simulink model "rtwdemo_capi"  (Simulink 7.6)
settings: Solver=FixedStepDiscrete  StartTime=0.0  StopTime=10.0  RelTol=1e-3  SampleTimeConstraint=STIndependent
PostLoadFcn:
  | rtwdemo_capi_data
values from neighbouring files (symbols this model uses):
  Kp = Simulink.Parameter    [rtwdemo_capi_data.m]
  p1 = Simulink.Parameter    [rtwdemo_capi_data.m]
  p2 = Simulink.Parameter    [rtwdemo_capi_data.m]
  p3 = Simulink.Parameter    [rtwdemo_capi_data.m]
libraries: rtwdemowidgets x2
Description:
  | Target-Based Data Interface: C-API Data Definition File
settings Model: Creator=The MathWorks Inc.  ExtModeTrigMode=oneshot  ExtModeArmWhenConnect=off  ExtModeAutoUpdateStatusClock=off
settings DataIOCC: LimitDataPoints=off  SaveFormat=Structure  SaveOutput=off  SaveTime=off  SignalLoggingName=sigsOut
settings OptimizationCC: InlineParams=on  InlineInvariantSignals=on  StateBitsets=on  DataBitsets=on  UseTempVars=on  EfficientFloat2IntCast=on
settings DebuggingCC: CheckExecutionContextPreStartOutputMsg=on  CheckExecutionContextRuntimeOutputMsg=on  SolverPrmCheckMsg=none  UnconnectedInputMsg=none  UnconnectedOutputMsg=none  UnconnectedLineMsg=none  ModelReferenceSymbolNameMessage=none  StrictBusMsg=ErrorOnBusTreatedAsVector
settings HardwareCC: ProdIntDivRoundTo=Zero  ProdEndianess=LittleEndian  ProdHWDeviceType=Generic->32-bit Embedded Processor  TargetHWDeviceType=Generic->32-bit Embedded Processor
settings RTWCC: TLCOptions=-p0 -aWarnNonSaturatedBlocks=0  GenerateReport=on  RTWVerbose=off  ProcessScript=grt_make_rtw_hook  LaunchReport=on
settings CodeAppCC: ForceParamTrailComments=on
settings GRTTargetCC: RTWCAPISignals=on  RTWCAPIParams=on  RTWCAPIStates=on

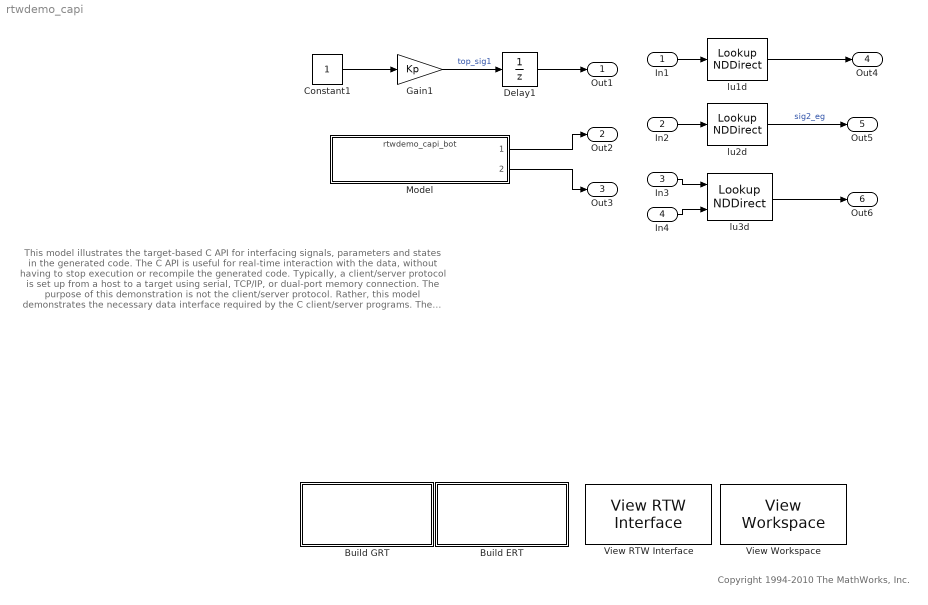
== system rtwdemo_capi ==
  note: This model illustrates the target-based C API for interfacing signals, parameters and states in the generated code.
      | The C API is useful for real-time interaction with the data, without having to stop execution or recompile the
      | generated code.  Typically, a client/server protocol is set up from a host to a target using serial, TCP/IP, or
      | dual-port memory connection.  The purpose of this demonstration is not the client/server protocol.  Rather,
      | this model demonstrates the necessary data interface required by the C client/server programs.
      |
      | The C-API is enabled by setting the Real-Time Workshop option "Data Exchange" to C API.  Any signal or
      | parameter or state with an addressable storage class is placed in the C API data structure in <model>_capi.c. Note
      | that signals, states and parameters in the referenced model can be accessed using C-API. So ensure that C-API is
      | enabled for the referenced model.
  note: Copyright 1994-2010 The MathWorks, Inc.
  In1 : Inport  OutDataTypeStr=double  PortDimensions=1
  In2 : Inport  Port=2  OutDataTypeStr=double  PortDimensions=1
  In3 : Inport  Port=3  OutDataTypeStr=double  PortDimensions=1
  In4 : Inport  Port=4  OutDataTypeStr=double  PortDimensions=1
  Build ERT : Subsystem  mask{attrib_overrides={'RTWCAPIParams','RTWCAPISignals','RTWCAPIStates'}}
      mask prompts: attrib_overrides "List of attributes to preserve (cell of strings):"
      mask help: Enter the attributes of the configuration set that you want preserved. Otherwise, the default configuration script will override your current settings.
      settings: OpenFcn=|
      | if ~exist('rtwdemo_ert', 'dir')
      |     disp('Creating working directory rtwdemo_ert')
      |     mkdir('rtwdemo_ert')
      | end
      | cd('rtwdemo_ert');
      | overrides=get_param(gcb,'attrib_overrides');
      | modelbot='rtwdemo_capi_bot';
      | load_system(modelbot);
      | ori_cs_bot = getActiveConfigSet(modelbot);
      | tmp_cs_bot = ori_cs_bot.copy;
      | tmp_cs_bot.Name = 'tempcs4bot';
      | attachConfigSet(modelbot, tmp_cs_bot);
      | setActiveConfigSet(modelbot, 'tempcs4bot');
      | rtwconfiguredemo(modelbot,'noop',false,overrides);
      | setProp(tmp_cs_bot,'CustomSymbolStr','$R$N$M');
      | set_param(modelbot,'dirty','off');
      | 
      | modeltop='rtwdemo_capi';
      | ori_cs_top=getActiveConfigSet(modeltop);
      | tmp_cs_top = ori_cs_top.copy;
      | tmp_cs_top.Name = 'tempcs4top';
      | attachConfigSet(modeltop, tmp_cs_top);
      | setActiveConfigSet(modeltop, 'tempcs4top');
      | 
      | rtwconfiguredemo(modeltop,'noop',false,overrides);
      | setProp(tmp_cs_top,'CustomSymbolStr','$R$N$M');
      | 
      | rtwbuilddemomodel(modeltop);
      | cd('..')
      | 
      | setActiveConfigSet(modelbot, ori_cs_bot.Name);
      | setActiveConfigSet(modeltop, ori_cs_top.Name);
      | tmp_cs_bot = detachConfigSet(modelbot, tmp_cs_bot.Name);
      | tmp_cs_top = detachConfigSet(modeltop, tmp_cs_top.Name);
      | 
      | set_param(modeltop,'dirty','off');
      | set_param(modelbot,'dirty','off');
      | close_system(modelbot);
      | 
      | clear modeltop modelbot overrides ori_cs_bot ori_cs_top tmp_cs_bot tmp_cs_top;
      mask Display:
      | disp(['Generate Code Using\n',...
      | 	  'Real-Time Workshop\n',...
      | 	  'Embedded Coder\n'...
      | 	  '(double-click)'])
  Build GRT : Subsystem  mask{attrib_overrides={'RTWCAPIParams','RTWCAPISignals','RTWCAPIStates'}}
      mask prompts: attrib_overrides "List of attributes to preserve (cell of strings):"
      mask help: Enter the attributes of the configuration set that you want preserved. Otherwise, the default configuration script will override your current settings.
      settings: OpenFcn=|
      | try
      |      if ~exist('rtwdemo_grt','dir')
      |          disp('Creating working directory rtwdemo_grt')
      |          mkdir('rtwdemo_grt');
      |      end
      |      chdir('rtwdemo_grt')
      |      overrides=get_param(gcb,'attrib_overrides');
      |      model='rtwdemo_capi_bot';
      |      load_system(model);
      |      rtwconfiguredemo(model,'noop',true,overrides);
      |      model='rtwdemo_capi';
      |      rtwconfiguredemo(model,'noop',true,overrides);
      |      rtwbuilddemomodel(model);
      |      cd('..');
      |  catch
      |      error(lasterr);
      |  end
      | 
      |  clear model overrides;
      mask Display:
      | disp(['Generate Code Using\n',...
      | 	  'Real-Time Workshop\n',...
      | 	  '(double-click)'])
  Constant1 : Constant
  Delay1 : UnitDelay  SampleTime=-1  StateIdentifier=top_state
  Gain1 : Gain  Gain=Kp  SaturateOnIntegerOverflow=on  OutDataTypeStr=Inherit: Same as input  ParamDataTypeStr=Inherit: Same as input
  Model : ModelReference  ModelNameDialog=rtwdemo_capi_bot  SimulationMode=Accelerator  ModelReferenceVersion=1.167  CopyOfModelName=rtwdemo_capi_bot
  View RTW Interface : rtwdemowidgets/View RTW Interface  SystemSampleTime=-1
  View Workspace : rtwdemowidgets/View Workspace  SystemSampleTime=-1
  lu1d : LookupNDDirect  Priority=5  NumberOfTableDimensions=1  Table=p1
  lu2d : LookupNDDirect  Priority=6  InputsSelectThisObjectFromTable=Column  Table=p2
  lu3d : LookupNDDirect  Priority=7  NumberOfTableDimensions=3  InputsSelectThisObjectFromTable=Column  Table=p3
  Out1 : Outport
  Out2 : Outport  Port=2
  Out3 : Outport  Port=3
  Out4 : Outport  Port=4
  Out5 : Outport  Port=5
  Out6 : Outport  Port=6
  wires:
  Gain1/1 -> Delay1/1  "top_sig1"
  Constant1/1 -> Gain1/1
  lu1d/1 -> Out4/1
  lu2d/1 -> Out5/1  "sig2_eg"
  lu3d/1 -> Out6/1
  In1/1 -> lu1d/1
  In2/1 -> lu2d/1
  In3/1 -> lu3d/1
  In4/1 -> lu3d/2
  Delay1/1 -> Out1/1
  Model/1 -> Out2/1
  Model/2 -> Out3/1

== system rtwdemo_capi/Build ERT ==

== system rtwdemo_capi/Build GRT ==
